simulink model "iap_host_demo"  (Simulink 7.3)
settings: Solver=FixedStepDiscrete  SolverMode=SingleTasking  StartTime=0.0  StopTime=10.0  RelTol=1e-3
PreLoadFcn:
  | waijung.modelPreload; % Required for working with Waijung Blockset. Do not remove.
undefined symbols (not defined in the file): A0, A1, A2, A3, A7, B0, B1, B10, B11, B12, B13, C1, C2, C3, C4, C5, HSEOSC, Link, LQFP176, ST, STM32F417IG
libraries: simulink x9, waijung_webserver_iap_lib x9, stm32f4_canbus_lib x4, waijung_webserver x3, stm32f4_device_config_lib x1
CloseFcn:
  | waijung.modelClose; % Required for working with Waijung Blockset. Do not remove.
settings Model: Creator=Krisada  LastModifiedBy=Krisada
settings OptimizationCC: OptimizeModelRefInitCode=on  LifeSpan=1
settings HardwareCC: ProdEndianess=LittleEndian  ProdHWDeviceType=ARM Compatible->Cortex - M4  TargetEndianess=LittleEndian  TargetHWDeviceType=ARM Compatible->Cortex - M4
settings RTWCC: SystemTargetFile=stm32f4.tlc  GenerateMakefile=off  TemplateMakefile=ert_default_tmf  Description=STM32F4 Target  ProcessScript=stm32f4_make_rtw_hook
settings CodeAppCC: IgnoreCustomStorageClasses=off
settings STFCustomTargetCC: ModelReferenceCompliant=off  CombineOutputUpdateFcns=on  ERTCustomFileBanners=on  SupportContinuousTime=off  SupportNonInlinedSFcns=off  SystemTargetFile=stm32f4.tlc
settings ERTTargetCC: MultiwordLength=2048  ModelReferenceCompliant=off  ParMdlRefBuildCompliant=off  CompOptLevelCompliant=off  ERTFirstTimeCompliant=off  ModelStepFunctionPrototypeControlCompliant=off  CPPClassGenCompliant=off  ExtModeMexFile=noextcomm  InlinedParameterPlacement=NonHierarchical  ERTSrcFileBannerTemplate=stm32f4_code_template.cgt  ERTHdrFileBannerTemplate=stm32f4_code_template.cgt  ERTDataSrcFileTemplate=stm32f4_code_template.cgt  ERTDataHdrFileTemplate=stm32f4_code_template.cgt  ERTCustomFileTemplate=stm32f4_file_process.tlc

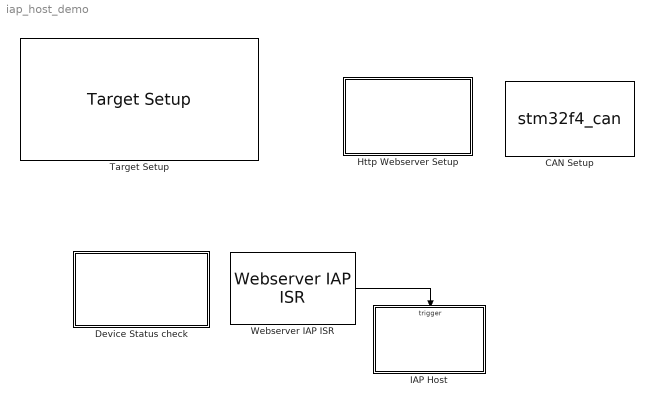
== system iap_host_demo ==
  CAN Setup : S-Function  FunctionName=stm32f4_can  Parameters=conf,canmodule,0,inputarray,outputarray,'','',confstr,sampletime,sampletimestr,blockid  EnableBusSupport=off  mask(stm32f4_can){conf=Setup, canmodule=1, advance=off, bitrate_select=125000, sjw=1tq, bs1=14tq, bs2=6tq, timingconf=Prescaler, brp=16, bitrate=125000, tq=3.8095e-007, remaptxpin=B9, remaprxpin=B8, sampletime=inf, sampletimestr=0.001, blockid=CANSetup, inputarray=[], inputlabelarray={}, outputarray=[], outputlabelarray={}, compat=0, confstr=["125000","16","B","9","B","8","1tq","14tq","6tq","ENABLE"], presc=16, txportstr=B, txpinstr=9, rxportstr=B, rxpinstr=8, lastmodule=1}
      mask prompts: conf "Configuration"; canmodule "CAN Module"; advance "Advance configuration"; bitrate_select "Baud rate (bps)"; sjw "Resync Jump Width (SJW)"; bs1 "Bit segment 1 (BS1) + PROP_SEG"; bs2 "Bit segment 2 (BS2)"; timingconf "Adjust"; brp "Baud rate prescaler (BRP)"; bitrate "Baud rate (bps)"; tq "Time Quantum (Second), tq"; remaptxpin "CAN Tx pin"; remaprxpin "CAN Rx pin"; sampletime "Sample time (sec)"; sampletimestr "Compiled sample time (sec) in string"; inputarray "Input port"; inputlabelarray "Input port label"; outputarray "Output port"; outputlabelarray "Output port label"; compat "Compatibility (Reserved for future use)"; confstr "Configuration String"; presc "Prescale"; txportstr "Tx port string"; txpinstr "Tx pin string"; rxportstr "Rx port string"; rxpinstr "Rx pin string"; lastmodule "Last module selected"
      mask help: This block setups CAN Module.
      mask init:
      | stm32f4_can_callback('init');
      mask Help: web(fullfile(waijungdocroot,'stm32f4_can_setup.htm'), '-browser')
      mask StyleString: popup(Setup),popup(1|2),checkbox,popup(125000|250000|500000|1000000),popup(1tq|2tq|3tq|4tq),popup(1tq|2tq|3tq|4tq|5tq|6tq|7tq|8tq|9tq|10tq|11tq|12tq|13tq|14tq|15tq|16tq),popup(1tq|2tq|3tq|4tq|5tq|6tq|7tq|8tq),popup(Prescaler|Baudrate),edit,edit,edit,popup(Not used|A12|B9|D1|H13),popup(Not used|A11|B8|D0|I9),edit,edit,edit,edit,edit,edit,edit,edit,edit,edit,edit,edit,edit,edit,edit
      mask CallbackString: |stm32f4_can_callback('canmodule');|stm32f4_can_callback('advance');|stm32f4_can_callback('bitrate_select');||stm32f4_can_callback('timingconf');|stm32f4_can_callback('timingconf');|stm32f4_can_callback('timingconf');|stm32f4_can_callback('timingconf');|stm32f4_can_callback('timingconf');||stm32f4_can_callback('remaptxpin');|stm32f4_can_callback('remaprxpin');|stm32f4_can_callback('sampletime');|stm32f4_can_callback('sampletimestr');|stm32f4_can_callback('blockid');||||||||||||
      mask Display: text(0.5, 0.5, 'CAN1_Setup\nSpeed (bps): 125000\nTx/Rx pin: B9/B8','ver','middle','hor','center');
  Device Status check : Subsystem  TreatAsAtomicUnit=on
  Http Webserver Setup : Subsystem
  IAP Host : Subsystem  TreatAsAtomicUnit=on
  Target Setup : stm32f4_device_config_lib/Target Setup  Priority=100  compiler=GNU ARM  previous_compiler=GNU ARM  mcu=STM32F417IG (LQFP176)  mcustr=STM32F417IG  clockconfig=HSEOSC-8MHz  system_stm32f4xx_c_path=F:\trunk\targets\stm32f4_target\stm32f4\utils\system_stm32f4xx_default\STM32F40_41xxx\hseosc8mhz  showmemoryconfiguration=off  stacksize=0x2000  heapsize=0x2000  enableautocompiledownload=on  fullchiperase=off  programmerinterface=ST-Link  editctrlstr=on  compilercontrolstr=$(patsubst %, -I%, .) -mcpu=cortex-m4 -mthumb -mthumb-interwork -mfloat-abi=hard -mfpu=fpv4-sp-d16 -ffast-math -Wall -Wextra -Ofast  assemblercontrolstr=$(patsubst %, -I%, .) -mcpu=cortex-m4 -mthumb -mthumb-interwork -mfloat-abi=hard -mfpu=fpv4-sp-d16 -ffast-math -Wall -Wextra -Ofast -Wa,-amhls=$(<:.s=.lst) -D__STACK_SIZE=$(STACK_SIZE) -D__HEAP_SIZE=$(HEAP_SIZE)  linkercontrolstr=-T$(LD_SCRIPT) -g -Wl,-Map=$(MAP),--cref,--no-warn-mismatch -mcpu=cortex-m4 -mthumb -mthumb-interwork -mfloat-abi=hard -mfpu=fpv4-sp-d16 -specs=nosys.specs  runafterdownload=on  execprofile=None  profileruart=3  profilerbaud=500000  profilertxpin=D8  profilerinitstr=0.001,168000000,168000,500000,0  manualsetsampletime=off  sampletime=0.001  blockid=TargetSetup  systickreloadvalue=168000  hseval=8000000  lastprofileruart=3  hclk=168000000  flashorigin=0x8000000  flashlength=1024k  ramorigin=0x20000000  ramlength=128k  useextram=off
  Webserver IAP ISR : waijung_webserver_iap_lib/Webserver IAP ISR  conf=ISR  enableisr=on  sampletime=inf  sampletimestr=Inf  blockid=WebserverIAPISR  inputarray=[]  inputlabelarray={}  outputarray=[7]  outputlabelarray={'Call ISR'}  compat=0  confstr="[\"Param1\",\"Param1\"]"
  wires:
  Webserver IAP ISR/1 -> IAP Host/Trigger

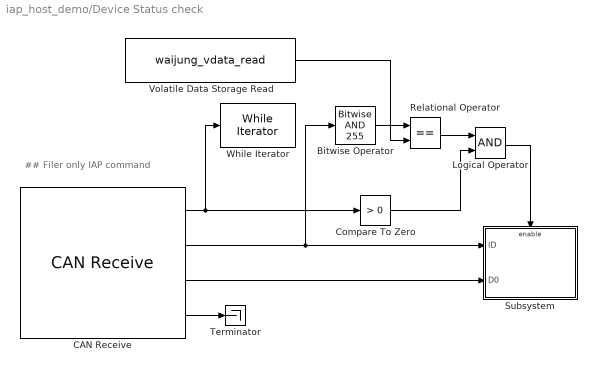
== system iap_host_demo/Device Status check ==
  note: ## Filer only IAP command
  Bitwise Operator : simulink/Logic and Bit Operations/Bitwise Operator  logicop=AND  UseBitMask=on  BitMask=255  BitMaskRealWorld=Stored Integer
  CAN Receive : stm32f4_canbus_lib/CAN Receive  conf=Rx  canmodule=1  idtype=Standard  filtertype=Mask  id=hex2dec('400')  idmask=hex2dec('4F0')  enableisr=off  usedlc=off  datatype=uint32  data0type=uint32  data1type=uint32  data2type=Not used  data3type=Not used  data4type=Not used  data5type=Not used  data6type=Not used  data7type=Not used  buffersize=32  sampletime=inf  sampletimestr=-1  blockid=DeviceStatuscheckCANReceive  inputarray=[]  inputlabelarray={}  outputarray=[ 5, 7, 7, 7]  outputlabelarray={ 'Msg Pending','ID', 'D0 (uint32)', 'D1 (uint32)' }  compat=0  confstr="[\"Standard\",\"Mask\",\"1024\",\"1264\",\"off\",\"uint32\",\"uint32\",\"Not used\",\"Not used\",\"Not used\",\"Not used\",\"Not used\",\"Not used\",\"32\",\"8000\",\"0\",\"9E00\",\"4\"]"
  Compare To Zero : simulink/Logic and Bit Operations/Compare To Zero  SystemSampleTime=-1  relop=>  LogicOutDataTypeMode=uint8  ZeroCross=off
  Logical Operator : Logic  AllPortsSameDT=off  OutDataTypeMode=boolean  LogicDataType=fixdt(0, 8)  OutDataTypeStr=boolean
  Relational Operator : RelationalOperator  Operator===  LogicOutDataTypeMode=boolean  LogicDataType=fixdt(0, 8)  OutDataTypeStr=boolean
  Subsystem : Subsystem
  Terminator : Terminator
  Volatile Data Storage Read : S-Function  FunctionName=waijung_vdata_read  Parameters=storagename,varname,sampletime,sampletimestr,blockid,storagetype,storagetypestr  EnableBusSupport=off  mask(waijung_vdata_read){storagename=IAP_Device_Id, varname=IAPHostVolatileDataStorage1_IAP_Device_Id, sampletime=inf, sampletimestr=-1, blockid=DeviceStatuscheckVolatileDataStorageRead, storagetype=uint32, storagetypestr=uint32_t}
      mask prompts: storagename "Storage Name"; varname "Variable name"; sampletime "Sample time (sec)"; sampletimestr "Compiled sample time (sec) in string"; storagetype "Data type"; storagetypestr "Data type string"
      mask help: This block implements read data from a buffer.
      mask init:
      | waijung_vdata_read_callback('init');
      mask Help: web(fullfile(waijungdocroot,'Volatile_Data_Storage_Read.htm'))
      mask StyleString: popup(IAP_Device_Id|IAP_Device_Sta),edit,edit,edit,edit,edit,edit
      mask CallbackString: waijung_vdata_read_callback('storagename');|waijung_vdata_read_callback('varname');|waijung_vdata_read_callback('sampletime');|waijung_vdata_read_callback('sampletimestr');|waijung_vdata_read_callback('blockid');|waijung_vdata_read_callback('storagetype');|
      mask Display: text(0.05, 0.5, 'Buffer: IAP_Device_Id','ver','middle','hor','left');port_label('output',1,'D1(uint32)')
  While Iterator : WhileIterator  WhileBlockType=do-while
  wires:
  CAN Receive/1 -> Compare To Zero/1, While Iterator/1
  CAN Receive/2 -> Subsystem/1(ID), Bitwise Operator/1
  CAN Receive/3 -> Subsystem/2(D0)
  Relational Operator/1 -> Logical Operator/1
  Compare To Zero/1 -> Logical Operator/2
  Logical Operator/1 -> Subsystem/Enable
  Bitwise Operator/1 -> Relational Operator/1
  Volatile Data Storage Read/1 -> Relational Operator/2
  CAN Receive/4 -> Terminator/1

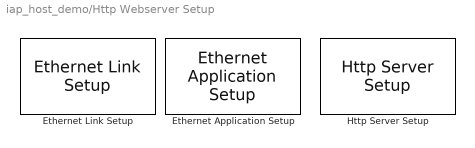
== system iap_host_demo/Http Webserver Setup ==
  Ethernet Application Setup : waijung_webserver/Ethernet Application Setup  conf=Setup  ipaddress=192.168.1.41  netmask=255.255.255.0  gateway=192.168.1.1  macaddress=02-00-00-00-00-00  dhcp=off  timerscaler=10  portpinstr=0  sampletime=0.001  blockid=HttpWebserverSetupEthernetApplicationSetup  inputporttype=[]  inputportwidth=[]  inputportlabel={}  outputporttype=[]  outputportwidth=[]  outputportlabel={}  compat=0  optionstring="[\"Dummy\",\"192\",\"168\",\"1\",\"41\",\"255\",\"255\",\"255\",\"0\",\"192\",\"168\",\"1\",\"1\",\"02\",\"00\",\"00\",\"00\",\"00\",\"00\",\"off\",\"10\"]"
  Ethernet Link Setup : waijung_webserver/Ethernet Link Setup  conf=Setup  interfacepin=Profile #1  wj_interfacetype=MII  pin_mdio=A2  pin_mdc=C1  pin_pps=Not used  pin_crs=A0  pin_col=A3  pin_dv=A7  pin_rxclk=A1  pin_rxer=B10  pin_rxd0=C4  pin_rxd1=C5  pin_rxd2=B0  pin_rxd3=B1  pin_txclk=C3  pin_txen=B11  pin_txd0=B12  pin_txd1=B13  pin_txd2=C2  pin_txd3=E2  portpinstr=A0,A1,A2,A3,A7,B0,B1,E2,B10,B11,B12,B13,C1,C2,C3,C4,C5  sampletime=inf  blockid=HttpWebserverSetupEthernetLinkSetup  inputporttype=[]  inputportwidth=[]  inputportlabel={}  outputporttype=[]  outputportwidth=[]  outputportlabel={}  compat=0  optionstring="[\"xxx\",\"on\",\"on\",\"on\",\"off\",\"on\",\"off\",\"off\",\"off\",\"off\",\"on\",\"on\",\"on\",\"on\",\"on\",\"on\",\"on\",\"off\",\"on\",\"on\",\"on\",\"on\",\"on\",\"on\",\"on\",\"on\",\"on\",\"on\",\"A\",\"0\",\"A\",\"1\",\"A\",\"2\",\"A\",\"3\",\"A\",\"7\",\"B\",\"0\",\"B\",\"1\",\"N\",\"ot used\",\"E\",\"2\",\"B\",\"10\",\"B\",\"11\",\"B\",\"12\",\"B\",\"13\",\"C\",\"1\",\"C\",\"2\",\"C\",\"3\",\"C\",\"4\",\"C\",\"5\",\"MII\"]"
  Http Server Setup : waijung_webserver/Http Server Setup  conf=Setup  port=80  ssl=Disable  sqlite=Disable  iap=Enable  mempool=8  debugport=Disable  portpinstr=0  sampletime=inf  blockid=HttpWebserverSetupHttpServerSetup  inputporttype=[]  inputportwidth=[]  inputportlabel={}  outputporttype=[]  outputportwidth=[]  outputportlabel={}  compat=0  optionstring="[\"80\",\"0\",\"0\",\"Disable\",\"Enable\",\"8\",\"17.02a\",\"\",\"\",\"\"]"

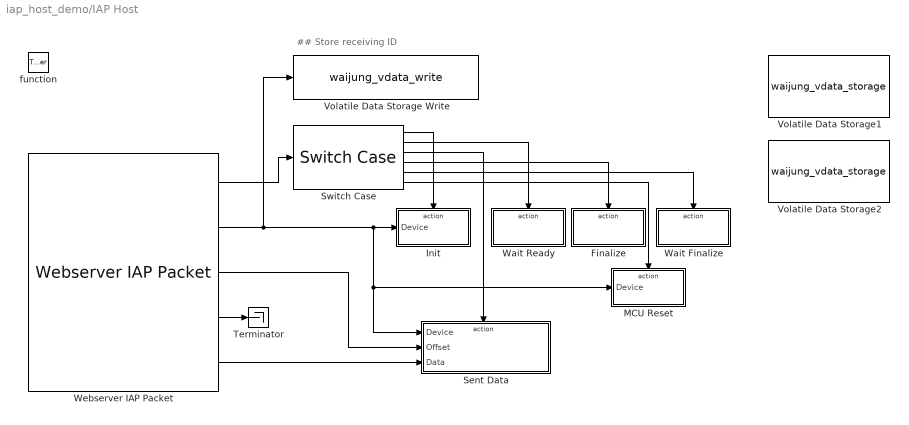
== system iap_host_demo/IAP Host ==
  note: ## Store receiving ID
  function : TriggerPort  TriggerType=function-call
  Finalize : Subsystem  TreatAsAtomicUnit=on
  Init : Subsystem  TreatAsAtomicUnit=on
  MCU Reset : Subsystem  TreatAsAtomicUnit=on
  Sent Data : Subsystem  TreatAsAtomicUnit=on
  Switch Case : SwitchCase  CaseConditions={0,1,2,3,4,5}  CaseShowDefault=off
  Terminator : Terminator
  Volatile Data Storage Write : S-Function  FunctionName=waijung_vdata_write  Parameters=storagename,varname,sampletime,sampletimestr,blockid,storagetype,storagetypestr  EnableBusSupport=off  mask(waijung_vdata_write){storagename=IAP_Device_Id, varname=IAPHostVolatileDataStorage1_IAP_Device_Id, sampletime=-1, sampletimestr=-1, blockid=IAPHostVolatileDataStorageWrite, storagetype=uint32, storagetypestr=uint32_t}
      mask prompts: storagename "Storage Name"; varname "Variable name"; sampletime "Sample time (sec)"; sampletimestr "Compiled sample time (sec) in string"; storagetype "Data type"; storagetypestr "Data type string"
      mask help: This block implements write data to a buffer.
      mask init:
      | waijung_vdata_write_callback('init');
      mask Help: web(fullfile(waijungdocroot,'Volatile_Data_Storage_Write.htm'))
      mask StyleString: popup(IAP_Device_Id|IAP_Device_Sta),edit,edit,edit,edit,edit,edit
      mask CallbackString: waijung_vdata_write_callback('storagename');|waijung_vdata_write_callback('varname');|waijung_vdata_write_callback('sampletime');|waijung_vdata_write_callback('sampletimestr');|waijung_vdata_write_callback('blockid');|waijung_vdata_write_callback('storagetype');|
      mask Display: text(0.95, 0.5, 'Buffer: IAP_Device_Id','ver','middle','hor','right');port_label('input',1,'D1(uint32)')
  Volatile Data Storage1 : S-Function  FunctionName=waijung_vdata_storage  Parameters=storagetype,storagename,initval,varname,buffersize,initvalstring,sampletime,sampletimestr,blockid,storagetypestr  EnableBusSupport=off  mask(waijung_vdata_storage){storagetype=uint32, storagename=IAP_Device_Id, initval=0, varname=IAPHostVolatileDataStorage1_IAP_Device_Id, buffersize=64, initvalstring='Initial string', webintegration=Disable, weboutputformat='%u', webcgicallback=(void*)0, laststoragetype=uint32, sampletime=-1, sampletimestr=-1, blockid=IAPHostVolatileDataStorage1, storagetypestr=uint32_t}
      mask prompts: storagetype "Storage Type"; storagename "Storage Name (must be a valid variable name)"; initval "Initial value (Apply at Power on Reset only)"; varname "Variable name"; buffersize "Size (bytes)"; initvalstring "Initial value (Apply at Power on Reset only)"; webintegration "Web CGI varget/varset integration"; weboutputformat "Web CGI varget output format"; webcgicallback "Web CGI varset callback"; laststoragetype "Last selected Storage Type"; sampletime "Sample time (sec)"; sampletimestr "Compiled sample time (sec) in string"; storagetypestr "Type string"
      mask help:
      | This block implements a volatile Data Storage.
      |
      | Web CGI varset/varget integratiopn:
      | Enable - In webserver application, allow remote access via http.
      | Disable - Variable is use in local only.
      mask init:
      | waijung_vdata_storage_callback('init');
      mask Help: web(fullfile(waijungdocroot,'Volatile_Data_Storage.htm'))
      mask StyleString: popup(double|single|uint32|int32|uint16|int16|uint8|int8|string),edit,edit,edit,edit,edit,popup(Disable|ReadOnly|Write/ Read|ReadOnly with KeyValuePair|Write/ Read with KeyValuePair),edit,edit,popup(double|single|uint32|int32|uint16|int16|uint8|int8|string),edit,edit,edit,edit
      mask CallbackString: waijung_vdata_storage_callback('storagetype');|waijung_vdata_storage_callback('storagename');|waijung_vdata_storage_callback('initval');|waijung_vdata_storage_callback('varname');||waijung_vdata_storage_callback('initvalstring');|waijung_vdata_storage_callback('webintegration');|waijung_vdata_storage_callback('weboutputformat');|||waijung_vdata_storage_callback('sampletime');|waijung_vdata_storage_callback('sampletimestr');|waijung_vdata_storage_callback('blockid');|
      mask Display: text(0.5, 0.5, 'Name: IAP_Device_Id\nType: uint32','ver','middle','hor','center')
  Volatile Data Storage2 : S-Function  FunctionName=waijung_vdata_storage  Parameters=storagetype,storagename,initval,varname,buffersize,initvalstring,sampletime,sampletimestr,blockid,storagetypestr  EnableBusSupport=off  mask(waijung_vdata_storage){storagetype=uint32, storagename=IAP_Device_Sta, initval=0, varname=IAPHostVolatileDataStorage2_IAP_Device_Sta, buffersize=64, initvalstring='Initial string', webintegration=Disable, weboutputformat='%u', webcgicallback=(void*)0, laststoragetype=uint32, sampletime=-1, sampletimestr=-1, blockid=IAPHostVolatileDataStorage2, storagetypestr=uint32_t}
      mask prompts: storagetype "Storage Type"; storagename "Storage Name (must be a valid variable name)"; initval "Initial value (Apply at Power on Reset only)"; varname "Variable name"; buffersize "Size (bytes)"; initvalstring "Initial value (Apply at Power on Reset only)"; webintegration "Web CGI varget/varset integration"; weboutputformat "Web CGI varget output format"; webcgicallback "Web CGI varset callback"; laststoragetype "Last selected Storage Type"; sampletime "Sample time (sec)"; sampletimestr "Compiled sample time (sec) in string"; storagetypestr "Type string"
      mask help:
      | This block implements a volatile Data Storage.
      |
      | Web CGI varset/varget integratiopn:
      | Enable - In webserver application, allow remote access via http.
      | Disable - Variable is use in local only.
      mask init:
      | waijung_vdata_storage_callback('init');
      mask Help: web(fullfile(waijungdocroot,'Volatile_Data_Storage.htm'))
      mask StyleString: popup(double|single|uint32|int32|uint16|int16|uint8|int8|string),edit,edit,edit,edit,edit,popup(Disable|ReadOnly|Write/ Read|ReadOnly with KeyValuePair|Write/ Read with KeyValuePair),edit,edit,popup(double|single|uint32|int32|uint16|int16|uint8|int8|string),edit,edit,edit,edit
      mask CallbackString: waijung_vdata_storage_callback('storagetype');|waijung_vdata_storage_callback('storagename');|waijung_vdata_storage_callback('initval');|waijung_vdata_storage_callback('varname');||waijung_vdata_storage_callback('initvalstring');|waijung_vdata_storage_callback('webintegration');|waijung_vdata_storage_callback('weboutputformat');|||waijung_vdata_storage_callback('sampletime');|waijung_vdata_storage_callback('sampletimestr');|waijung_vdata_storage_callback('blockid');|
      mask Display: text(0.5, 0.5, 'Name: IAP_Device_Sta\nType: uint32','ver','middle','hor','center')
  Wait Finalize : Subsystem  TreatAsAtomicUnit=on
  Wait Ready : Subsystem  TreatAsAtomicUnit=on
  Webserver IAP Packet : waijung_webserver_iap_lib/Webserver IAP Packet  conf=Packet  enableisr=off  sampletime=inf  sampletimestr=-1  blockid=IAPHostWebserverIAPPacket  inputarray=[]  inputlabelarray={}  outputarray=[7,7,7,7,7]  outputlabelarray={'State','Device','Data Offset','Data Size (Total)','Data (uint32)'}  compat=0  confstr="[\"Param1\",\"Param1\"]"
  wires:
  Webserver IAP Packet/1 -> Switch Case/1
  Switch Case/1 -> Init/Action
  Switch Case/2 -> Wait Ready/Action
  Switch Case/3 -> Sent Data/Action
  Switch Case/4 -> Finalize/Action
  Switch Case/5 -> Wait Finalize/Action
  Switch Case/6 -> MCU Reset/Action
  Webserver IAP Packet/2 -> Volatile Data Storage Write/1, Init/1(Device), Sent Data/1(Device), MCU Reset/1(Device)
  Webserver IAP Packet/3 -> Sent Data/2(Offset)
  Webserver IAP Packet/4 -> Terminator/1
  Webserver IAP Packet/5 -> Sent Data/3(Data)

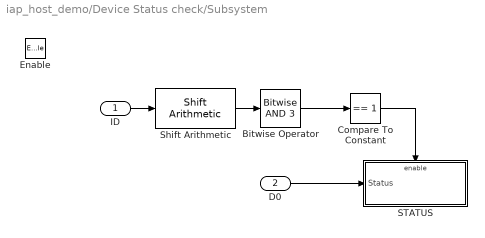
== system iap_host_demo/Device Status check/Subsystem ==
  ID : Inport
  D0 : Inport  Port=2
  Enable : EnablePort
  Bitwise Operator : simulink/Logic and Bit Operations/Bitwise Operator  logicop=AND  UseBitMask=on  BitMask=3  BitMaskRealWorld=Stored Integer
  Compare To Constant : simulink/Logic and Bit Operations/Compare To Constant  SystemSampleTime=-1  relop===  const=1  LogicOutDataTypeMode=uint8  ZeroCross=off
  STATUS : Subsystem  TreatAsAtomicUnit=on
  Shift Arithmetic : simulink/Logic and Bit Operations/Shift Arithmetic  SystemSampleTime=-1  nBitShiftRight=8  nBinPtShiftRight=0
  wires:
  Shift Arithmetic/1 -> Bitwise Operator/1
  Bitwise Operator/1 -> Compare To Constant/1
  Compare To Constant/1 -> STATUS/Enable
  ID/1 -> Shift Arithmetic/1
  D0/1 -> STATUS/1(Status)

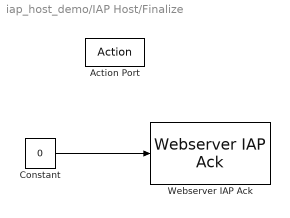
== system iap_host_demo/IAP Host/Finalize ==
  Action Port : ActionPort  ActionType=case
  Constant : Constant  Value=0  OutDataType=fixdt(1, 16)  OutScaling=2^0
  Webserver IAP Ack : waijung_webserver_iap_lib/Webserver IAP Ack  conf=Ack  enableisr=off  sampletime=inf  sampletimestr=-1  blockid=IAPHostFinalizeWebserverIAPAck  inputarray=[-1]  inputlabelarray={'Status'}  outputarray=[]  outputlabelarray={}  compat=0  confstr="[\"Param1\",\"Param1\"]"
  wires:
  Constant/1 -> Webserver IAP Ack/1

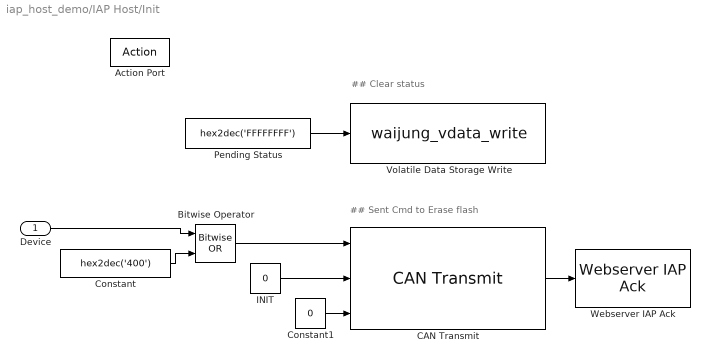
== system iap_host_demo/IAP Host/Init ==
  note: ## Sent Cmd to Erase flash
  note: ## Clear status
  Device : Inport  OutDataType=fixdt(1, 16)  OutScaling=2^0
  Action Port : ActionPort  ActionType=case
  Bitwise Operator : simulink/Logic and Bit Operations/Bitwise Operator  logicop=OR  UseBitMask=off  NumInputPorts=2  BitMask=bin2dec('11011001')  BitMaskRealWorld=Stored Integer
  CAN Transmit : stm32f4_canbus_lib/CAN Transmit  conf=Tx  canmodule=1  transfer=Blocking  timeout=0.005  idtype=Standard  specificid=off  id=0  specificdlc=on  dlc=8  enablestatus=on  datatype=uint32  data0type=uint32  data1type=uint32  data2type=Not used  data3type=Not used  data4type=Not used  data5type=Not used  data6type=Not used  data7type=Not used  inputarray=[ -1, 7, 7]  inputlabelarray={ 'ID', 'D0 (uint32)', 'D1 (uint32)' }  outputarray=[7]  outputlabelarray={'Status'}  sampletime=-1  sampletimestr=-1  blockid=IAPHostInitCANTransmit  compat=0  confstr="[\"Blocking\",\"0.005\",\"Standard\",\"off\",\"0\",\"on\",\"8\",\"on\",\"uint32\",\"uint32\",\"Not used\",\"Not used\",\"Not used\",\"Not used\",\"Not used\",\"Not used\"]"
  Constant : Constant  Value=hex2dec('400')  OutDataTypeMode=uint32  OutDataType=fixdt(1, 16)  OutScaling=2^0  OutDataTypeStr=uint32
  Constant1 : Constant  Value=0  OutDataTypeMode=uint32  OutDataType=fixdt(1, 16)  OutScaling=2^0  OutDataTypeStr=uint32
  INIT : Constant  Value=0  OutDataTypeMode=uint32  OutDataType=fixdt(1, 16)  OutScaling=2^0  OutDataTypeStr=uint32
  Pending Status : Constant  Value=hex2dec('FFFFFFFF')  OutDataTypeMode=uint32  OutDataType=fixdt(1, 16)  OutScaling=2^0  OutDataTypeStr=uint32
  Volatile Data Storage Write : S-Function  FunctionName=waijung_vdata_write  Parameters=storagename,varname,sampletime,sampletimestr,blockid,storagetype,storagetypestr  EnableBusSupport=off  mask(waijung_vdata_write){storagename=IAP_Device_Sta, varname=IAPHostVolatileDataStorage2_IAP_Device_Sta, sampletime=-1, sampletimestr=-1, blockid=IAPHostInitVolatileDataStorageWrite, storagetype=uint32, storagetypestr=uint32_t}
      mask prompts: storagename "Storage Name"; varname "Variable name"; sampletime "Sample time (sec)"; sampletimestr "Compiled sample time (sec) in string"; storagetype "Data type"; storagetypestr "Data type string"
      mask help: This block implements write data to a buffer.
      mask init:
      | waijung_vdata_write_callback('init');
      mask Help: web(fullfile(waijungdocroot,'Volatile_Data_Storage_Write.htm'))
      mask StyleString: popup(IAP_Device_Id|IAP_Device_Sta),edit,edit,edit,edit,edit,edit
      mask CallbackString: waijung_vdata_write_callback('storagename');|waijung_vdata_write_callback('varname');|waijung_vdata_write_callback('sampletime');|waijung_vdata_write_callback('sampletimestr');|waijung_vdata_write_callback('blockid');|waijung_vdata_write_callback('storagetype');|
      mask Display: text(0.95, 0.5, 'Buffer: IAP_Device_Sta','ver','middle','hor','right');port_label('input',1,'D1(uint32)')
  Webserver IAP Ack : waijung_webserver_iap_lib/Webserver IAP Ack  conf=Ack  enableisr=off  sampletime=inf  sampletimestr=-1  blockid=IAPHostInitWebserverIAPAck  inputarray=[-1]  inputlabelarray={'Status'}  outputarray=[]  outputlabelarray={}  compat=0  confstr="[\"Param1\",\"Param1\"]"
  wires:
  Device/1 -> Bitwise Operator/1
  Constant/1 -> Bitwise Operator/2
  Bitwise Operator/1 -> CAN Transmit/1
  Constant1/1 -> CAN Transmit/3
  INIT/1 -> CAN Transmit/2
  CAN Transmit/1 -> Webserver IAP Ack/1
  Pending Status/1 -> Volatile Data Storage Write/1

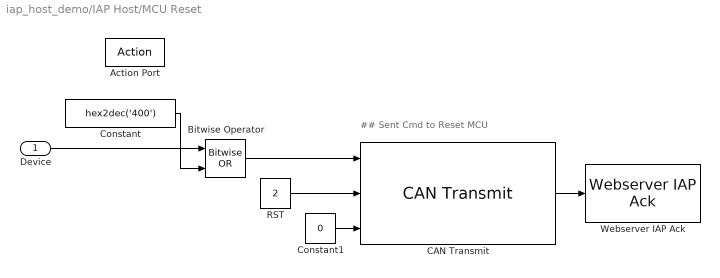
== system iap_host_demo/IAP Host/MCU Reset ==
  note: ## Sent Cmd to Reset MCU
  Device : Inport  OutDataType=fixdt(1, 16)  OutScaling=2^0
  Action Port : ActionPort  ActionType=case
  Bitwise Operator : simulink/Logic and Bit Operations/Bitwise Operator  logicop=OR  UseBitMask=off  NumInputPorts=2  BitMask=bin2dec('11011001')  BitMaskRealWorld=Stored Integer
  CAN Transmit : stm32f4_canbus_lib/CAN Transmit  conf=Tx  canmodule=1  transfer=Blocking  timeout=0.005  idtype=Standard  specificid=off  id=0  specificdlc=on  dlc=8  enablestatus=on  datatype=uint32  data0type=uint32  data1type=uint32  data2type=Not used  data3type=Not used  data4type=Not used  data5type=Not used  data6type=Not used  data7type=Not used  inputarray=[ -1, 7, 7]  inputlabelarray={ 'ID', 'D0 (uint32)', 'D1 (uint32)' }  outputarray=[7]  outputlabelarray={'Status'}  sampletime=-1  sampletimestr=-1  blockid=IAPHostMCUResetCANTransmit  compat=0  confstr="[\"Blocking\",\"0.005\",\"Standard\",\"off\",\"0\",\"on\",\"8\",\"on\",\"uint32\",\"uint32\",\"Not used\",\"Not used\",\"Not used\",\"Not used\",\"Not used\",\"Not used\"]"
  Constant : Constant  Value=hex2dec('400')  OutDataTypeMode=uint32  OutDataType=fixdt(1, 16)  OutScaling=2^0  OutDataTypeStr=uint32
  Constant1 : Constant  Value=0  OutDataTypeMode=uint32  OutDataType=fixdt(1, 16)  OutScaling=2^0  OutDataTypeStr=uint32
  RST : Constant  Value=2  OutDataTypeMode=uint32  OutDataType=fixdt(1, 16)  OutScaling=2^0  OutDataTypeStr=uint32
  Webserver IAP Ack : waijung_webserver_iap_lib/Webserver IAP Ack  conf=Ack  enableisr=off  sampletime=inf  sampletimestr=-1  blockid=IAPHostMCUResetWebserverIAPAck  inputarray=[-1]  inputlabelarray={'Status'}  outputarray=[]  outputlabelarray={}  compat=0  confstr="[\"Param1\",\"Param1\"]"
  wires:
  Device/1 -> Bitwise Operator/1
  Constant/1 -> Bitwise Operator/2
  Bitwise Operator/1 -> CAN Transmit/1
  Constant1/1 -> CAN Transmit/3
  RST/1 -> CAN Transmit/2
  CAN Transmit/1 -> Webserver IAP Ack/1

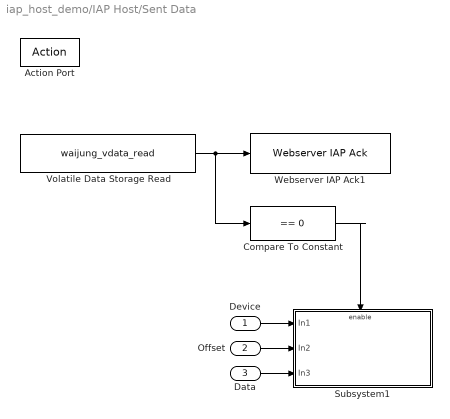
== system iap_host_demo/IAP Host/Sent Data ==
  Device : Inport  OutDataType=fixdt(1, 16)  OutScaling=2^0
  Offset : Inport  Port=2  OutDataType=fixdt(1, 16)  OutScaling=2^0
  Data : Inport  Port=3  OutDataType=fixdt(1, 16)  OutScaling=2^0
  Action Port : ActionPort  ActionType=case
  Compare To Constant : simulink/Logic and Bit Operations/Compare To Constant  SystemSampleTime=-1  relop===  const=0  LogicOutDataTypeMode=uint8  ZeroCross=off
  Subsystem1 : Subsystem
  Volatile Data Storage Read : S-Function  FunctionName=waijung_vdata_read  Parameters=storagename,varname,sampletime,sampletimestr,blockid,storagetype,storagetypestr  EnableBusSupport=off  mask(waijung_vdata_read){storagename=IAP_Device_Sta, varname=IAPHostVolatileDataStorage2_IAP_Device_Sta, sampletime=inf, sampletimestr=-1, blockid=IAPHostSentDataVolatileDataStorageRead, storagetype=uint32, storagetypestr=uint32_t}
      mask prompts: storagename "Storage Name"; varname "Variable name"; sampletime "Sample time (sec)"; sampletimestr "Compiled sample time (sec) in string"; storagetype "Data type"; storagetypestr "Data type string"
      mask help: This block implements read data from a buffer.
      mask init:
      | waijung_vdata_read_callback('init');
      mask Help: web(fullfile(waijungdocroot,'Volatile_Data_Storage_Read.htm'))
      mask StyleString: popup(IAP_Device_Id|IAP_Device_Sta),edit,edit,edit,edit,edit,edit
      mask CallbackString: waijung_vdata_read_callback('storagename');|waijung_vdata_read_callback('varname');|waijung_vdata_read_callback('sampletime');|waijung_vdata_read_callback('sampletimestr');|waijung_vdata_read_callback('blockid');|waijung_vdata_read_callback('storagetype');|
      mask Display: text(0.05, 0.5, 'Buffer: IAP_Device_Sta','ver','middle','hor','left');port_label('output',1,'D1(uint32)')
  Webserver IAP Ack1 : waijung_webserver_iap_lib/Webserver IAP Ack  conf=Ack  enableisr=off  sampletime=inf  sampletimestr=-1  blockid=IAPHostSentDataWebserverIAPAck1  inputarray=[-1]  inputlabelarray={'Status'}  outputarray=[]  outputlabelarray={}  compat=0  confstr="[\"Param1\",\"Param1\"]"
  wires:
  Device/1 -> Subsystem1/1(In1)
  Offset/1 -> Subsystem1/2(In2)
  Data/1 -> Subsystem1/3(In3)
  Volatile Data Storage Read/1 -> Webserver IAP Ack1/1, Compare To Constant/1
  Compare To Constant/1 -> Subsystem1/Enable

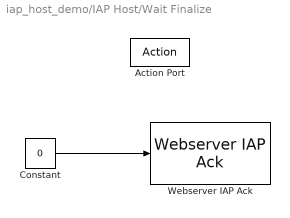
== system iap_host_demo/IAP Host/Wait Finalize ==
  Action Port : ActionPort  ActionType=case
  Constant : Constant  Value=0  OutDataType=fixdt(1, 16)  OutScaling=2^0
  Webserver IAP Ack : waijung_webserver_iap_lib/Webserver IAP Ack  conf=Ack  enableisr=off  sampletime=inf  sampletimestr=-1  blockid=IAPHostWaitFinalizeWebserverIAPAck  inputarray=[-1]  inputlabelarray={'Status'}  outputarray=[]  outputlabelarray={}  compat=0  confstr="[\"Param1\",\"Param1\"]"
  wires:
  Constant/1 -> Webserver IAP Ack/1

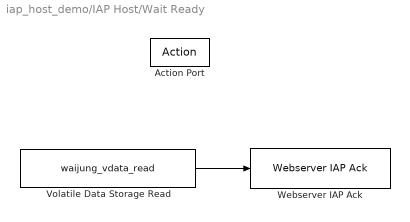
== system iap_host_demo/IAP Host/Wait Ready ==
  Action Port : ActionPort  ActionType=case
  Volatile Data Storage Read : S-Function  FunctionName=waijung_vdata_read  Parameters=storagename,varname,sampletime,sampletimestr,blockid,storagetype,storagetypestr  EnableBusSupport=off  mask(waijung_vdata_read){storagename=IAP_Device_Sta, varname=IAPHostVolatileDataStorage2_IAP_Device_Sta, sampletime=inf, sampletimestr=-1, blockid=IAPHostWaitReadyVolatileDataStorageRead, storagetype=uint32, storagetypestr=uint32_t}
      mask prompts: storagename "Storage Name"; varname "Variable name"; sampletime "Sample time (sec)"; sampletimestr "Compiled sample time (sec) in string"; storagetype "Data type"; storagetypestr "Data type string"
      mask help: This block implements read data from a buffer.
      mask init:
      | waijung_vdata_read_callback('init');
      mask Help: web(fullfile(waijungdocroot,'Volatile_Data_Storage_Read.htm'))
      mask StyleString: popup(IAP_Device_Id|IAP_Device_Sta),edit,edit,edit,edit,edit,edit
      mask CallbackString: waijung_vdata_read_callback('storagename');|waijung_vdata_read_callback('varname');|waijung_vdata_read_callback('sampletime');|waijung_vdata_read_callback('sampletimestr');|waijung_vdata_read_callback('blockid');|waijung_vdata_read_callback('storagetype');|
      mask Display: text(0.05, 0.5, 'Buffer: IAP_Device_Sta','ver','middle','hor','left');port_label('output',1,'D1(uint32)')
  Webserver IAP Ack : waijung_webserver_iap_lib/Webserver IAP Ack  conf=Ack  enableisr=off  sampletime=inf  sampletimestr=-1  blockid=IAPHostWaitReadyWebserverIAPAck  inputarray=[-1]  inputlabelarray={'Status'}  outputarray=[]  outputlabelarray={}  compat=0  confstr="[\"Param1\",\"Param1\"]"
  wires:
  Volatile Data Storage Read/1 -> Webserver IAP Ack/1

== system iap_host_demo/Device Status check/Subsystem/STATUS ==
  Status : Inport  OutDataType=fixdt(1, 16)  OutScaling=2^0
  Enable : EnablePort
  Volatile Data Storage Write : S-Function  FunctionName=waijung_vdata_write  Parameters=storagename,varname,sampletime,sampletimestr,blockid,storagetype,storagetypestr  EnableBusSupport=off  mask(waijung_vdata_write){storagename=IAP_Device_Sta, varname=IAPHostVolatileDataStorage2_IAP_Device_Sta, sampletime=-1, sampletimestr=-1, blockid=DeviceStatuscheckSubsystemSTATUSVolatileDataStorageWrite, storagetype=uint32, storagetypestr=uint32_t}
      mask prompts: storagename "Storage Name"; varname "Variable name"; sampletime "Sample time (sec)"; sampletimestr "Compiled sample time (sec) in string"; storagetype "Data type"; storagetypestr "Data type string"
      mask help: This block implements write data to a buffer.
      mask init:
      | waijung_vdata_write_callback('init');
      mask Help: web(fullfile(waijungdocroot,'Volatile_Data_Storage_Write.htm'))
      mask StyleString: popup(IAP_Device_Id|IAP_Device_Sta),edit,edit,edit,edit,edit,edit
      mask CallbackString: waijung_vdata_write_callback('storagename');|waijung_vdata_write_callback('varname');|waijung_vdata_write_callback('sampletime');|waijung_vdata_write_callback('sampletimestr');|waijung_vdata_write_callback('blockid');|waijung_vdata_write_callback('storagetype');|
      mask Display: text(0.95, 0.5, 'Buffer: IAP_Device_Sta','ver','middle','hor','right');port_label('input',1,'D1(uint32)')
  wires:
  Status/1 -> Volatile Data Storage Write/1

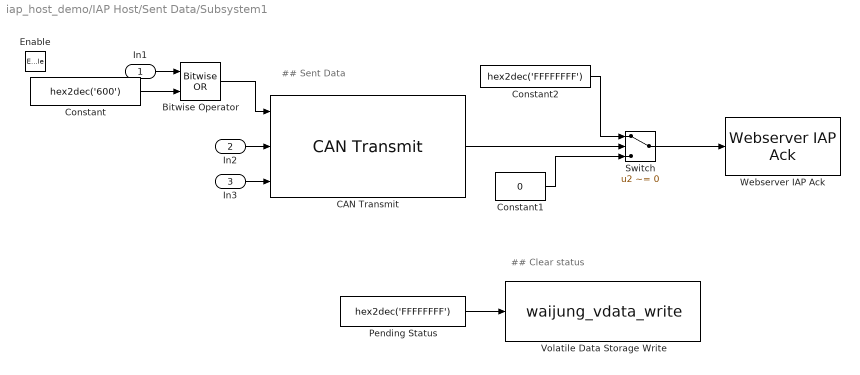
== system iap_host_demo/IAP Host/Sent Data/Subsystem1 ==
  note: ## Sent Data
  note: ## Clear status
  In1 : Inport
  In2 : Inport  Port=2
  In3 : Inport  Port=3
  Enable : EnablePort
  Bitwise Operator : simulink/Logic and Bit Operations/Bitwise Operator  logicop=OR  UseBitMask=off  NumInputPorts=2  BitMask=bin2dec('11011001')  BitMaskRealWorld=Stored Integer
  CAN Transmit : stm32f4_canbus_lib/CAN Transmit  conf=Tx  canmodule=1  transfer=Blocking  timeout=0.01  idtype=Standard  specificid=off  id=0  specificdlc=on  dlc=8  enablestatus=on  datatype=uint32  data0type=uint32  data1type=uint32  data2type=Not used  data3type=Not used  data4type=Not used  data5type=Not used  data6type=Not used  data7type=Not used  inputarray=[ -1, 7, 7]  inputlabelarray={ 'ID', 'D0 (uint32)', 'D1 (uint32)' }  outputarray=[7]  outputlabelarray={'Status'}  sampletime=-1  sampletimestr=-1  blockid=IAPHostSentDataSubsystem1CANTransmit  compat=0  confstr="[\"Blocking\",\"0.01\",\"Standard\",\"off\",\"0\",\"on\",\"8\",\"on\",\"uint32\",\"uint32\",\"Not used\",\"Not used\",\"Not used\",\"Not used\",\"Not used\",\"Not used\"]"
  Constant : Constant  Value=hex2dec('600')  OutDataTypeMode=uint32  OutDataType=fixdt(1, 16)  OutScaling=2^0  OutDataTypeStr=uint32
  Constant1 : Constant  Value=0  OutDataTypeMode=uint32  OutDataType=fixdt(1, 16)  OutScaling=2^0  OutDataTypeStr=uint32
  Constant2 : Constant  Value=hex2dec('FFFFFFFF')  OutDataTypeMode=uint32  OutDataType=fixdt(1, 16)  OutScaling=2^0  OutDataTypeStr=uint32
  Pending Status : Constant  Value=hex2dec('FFFFFFFF')  OutDataTypeMode=uint32  OutDataType=fixdt(1, 16)  OutScaling=2^0  OutDataTypeStr=uint32
  Switch : Switch  Criteria=u2 ~= 0  OutDataType=fixdt(1, 16)  OutScaling=2^0
  Volatile Data Storage Write : S-Function  FunctionName=waijung_vdata_write  Parameters=storagename,varname,sampletime,sampletimestr,blockid,storagetype,storagetypestr  EnableBusSupport=off  mask(waijung_vdata_write){storagename=IAP_Device_Sta, varname=IAPHostVolatileDataStorage2_IAP_Device_Sta, sampletime=-1, sampletimestr=-1, blockid=IAPHostSentDataSubsystem1VolatileDataStorageWrite, storagetype=uint32, storagetypestr=uint32_t}
      mask prompts: storagename "Storage Name"; varname "Variable name"; sampletime "Sample time (sec)"; sampletimestr "Compiled sample time (sec) in string"; storagetype "Data type"; storagetypestr "Data type string"
      mask help: This block implements write data to a buffer.
      mask init:
      | waijung_vdata_write_callback('init');
      mask Help: web(fullfile(waijungdocroot,'Volatile_Data_Storage_Write.htm'))
      mask StyleString: popup(IAP_Device_Id|IAP_Device_Sta),edit,edit,edit,edit,edit,edit
      mask CallbackString: waijung_vdata_write_callback('storagename');|waijung_vdata_write_callback('varname');|waijung_vdata_write_callback('sampletime');|waijung_vdata_write_callback('sampletimestr');|waijung_vdata_write_callback('blockid');|waijung_vdata_write_callback('storagetype');|
      mask Display: text(0.95, 0.5, 'Buffer: IAP_Device_Sta','ver','middle','hor','right');port_label('input',1,'D1(uint32)')
  Webserver IAP Ack : waijung_webserver_iap_lib/Webserver IAP Ack  conf=Ack  enableisr=off  sampletime=inf  sampletimestr=-1  blockid=IAPHostSentDataSubsystem1WebserverIAPAck  inputarray=[-1]  inputlabelarray={'Status'}  outputarray=[]  outputlabelarray={}  compat=0  confstr="[\"Param1\",\"Param1\"]"
  wires:
  Constant/1 -> Bitwise Operator/2
  Bitwise Operator/1 -> CAN Transmit/1
  CAN Transmit/1 -> Switch/2
  Constant1/1 -> Switch/3
  Constant2/1 -> Switch/1
  Switch/1 -> Webserver IAP Ack/1
  In1/1 -> Bitwise Operator/1
  In2/1 -> CAN Transmit/2
  In3/1 -> CAN Transmit/3
  Pending Status/1 -> Volatile Data Storage Write/1
